simulink library "PTOSim_Lib_UpdatedV3"  (R2020b)
settings: Solver=ode45  StartTime=0.0  StopTime=10.0  RelTol=1e-3  EnableMultiTasking=on
undefined symbols (not defined in the file or in its folder): DiscIntNeverNeededParam, ptosim, PTOSimBlock, simu
libraries: $bdroot x6
(part 1 of 2)
settings Model: RequirementInfo="{}  %GIDa_42666abb_d6d9_408c_ae24_f6520282b61c"  Creator=sor  LastModifiedBy=jleonqu
settings DataIOCC: LimitDataPoints=on  SaveFormat=Array  ReturnWorkspaceOutputs=off
settings OptimizationCC: LifeSpan=inf
settings DebuggingCC: SolverPrmCheckMsg=warning  AllowSymbolicDim=off  SFUnexpectedBacktrackingDiag=warning  SFNoUnconditionalDefaultTransitionDiag=warning  SFExecutionAtInitializationDiag=none  ArithmeticOperatorsInVariantConditions=warning
settings HardwareCC: ProdBitPerPointer=32  ProdBitPerSizeT=32  ProdBitPerPtrDiffT=32  ProdLargestAtomicFloat=None  ProdIntDivRoundTo=Undefined  ProdEndianess=Unspecified  ProdWordSize=32  ProdHWDeviceType=32-bit Generic
settings ModelReferenceCC: PropagateSignalLabelsOutOfModel=off
settings SFSimCC: SimUseLocalCustomCode=off  CustomCodeUndefinedFunction=UseInterfaceOnly
settings RTWCC: RTWUseLocalCustomCode=off
settings CodeAppCC: StateflowObjectComments=on
settings GRTTargetCC: TargetLangStandard=C89/C90 (ANSI)
settings ConfigComp: CovMetricSettings=dw  CovSaveCumulativeToWorkspaceVar=on  CovSaveSingleToWorkspaceVar=on  CovExternalEMLEnable=off  CovSFcnEnable=off

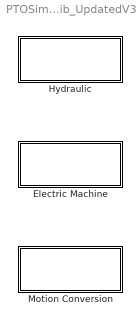
== system PTOSim_Lib_UpdatedV3 ==
  Electric Machine : Subsystem  RequirementInfo="{}  %GIDa_5439fdb4_7c29_433c_8677_23bf92e18f11"
  Hydraulic : Subsystem  RequirementInfo={} %GIDa_f12a42eb_b9cb_4818_b573_b7dee4183a3b
  Motion Conversion : Subsystem

== system PTOSim_Lib_UpdatedV3/Electric Machine ==
  Electric Machine Equivalent Circuit : Subsystem  mask{PTOSimBlock=PTOSimBlock(1), InputFiletext=Use PTO-Sim input file to define Electric Machine parameters, Ra=0, La=0, Ke=0, bShaft=0, Jem=0}
      mask prompts: PTOSimBlock "Electric Machine Name"; Ra "Armature Resistance [ohm]"; La "Armature Inductance [H]"; Ke "Back-emf or Torque constant [V/(rad/s)]"; bShaft "Rotor Damping [N s/m]"; Jem "Rotor Inertia [kg m^2]"
      mask init:
      | if exist('PTOSimBlock','var')
      |     h=[gcb '/To Workspace'];
      |     responseName=['PTOSimBlock' num2str(PTOSimBlock.PTOSimBlockNum) '_out'];
      |     set_param(h,'VariableName',responseName);
      | end
      | clear h responseName
      | %HydraulicBlock.checkLoc('W');
      settings: PortSchema="{\"entries\":[{\"content\":{\"sides\":[{\"content\":{\"connectorIds\":[\"In1\"]},\"type\":\"ConnectorPlacement.EquallySpacedRectSide\",\"uuid\":\"38b15b7d-d952-45b6-9eb0-5d473736364e\"},{\"content\":{\"connectorIds\":[\"Out1\"],\"side\":\"RIGHT\"},\"type\":\"ConnectorPlacement.EquallySpacedRectSide\",\"uuid\":\"de64adb9-f2de-4dd5-b519-c63af884483d\"},{\"content\":{\"connectorIds\":[\"In2\"],\"side\":\"TOP\"},\"type\":\"ConnectorPlacement.EquallySpacedRectSide\",\"uuid\":\"eaa9506a-5e37-41b4-975c-a8d526700d36\"},{\"content\":{\"connectorIds\":[],\"side\":\"HIDDEN\"},\"type\":\"ConnectorPlacement.EquallySpacedRectSide\",\"uuid\":\"f8da1221-e5bc-4844-b966-beaaa1d6bf60\"}]},\"type\":\"ConnectorPlacement.EquallySpacedConnector\",\"uuid\":\"4da2b473-e94d-42dc-9143-64fbcbf5d9e1\"}],\"packageUris\":[\"http://schema.mathworks.com/mf0/Connector/R2020b\"],\"version\":\"1.0\"}"
      mask DialogControl ParameterGroupVar Prompt: Custom Parameters
      mask DialogControl EMParameters Prompt: Electric Machine Parameters
      mask Display: image('ElectricMotor.png'); % Use "Edit Image" on toolstrip to change.

== system PTOSim_Lib_UpdatedV3/Hydraulic ==
  Compressible Fluid Piston Updated : Subsystem  mask{PTOSimBlock=PTOSimBlock(1), InputFileText=Use PTO-Sim input file to define PTO parameters, Ap_A=0, Ap_B=0, PistonStroke=0, BulkModulus=0, xi_piston=0, pAi=0, pBi=0}
      mask prompts: PTOSimBlock "Piston Name"; Ap_A "Piston area A [m]"; Ap_B "Piston area B [m]"; PistonStroke "Piston stroke [m]"; BulkModulus "Fluid Bulk Modulus [Pa]"; xi_piston "Piston initial displacement from A [m]"; pAi "Port A Initial pressure [Pa]"; pBi "Port B Initial pressure [Pa]"
      mask help:
      | PTO-Sim Compressible Fluid Piston
      |
      | This block simualtes a hydraulic cylinder using a compressible fluid model. The block inputs are Response and HydraulicInput. Response is the signal output of the block Rotational PTO Actuation Force. HydraulicInput is a two signal vector with the information of the flow rate for port A and port B of the cylinder. The output of the block is PistonOutput, which is a three signal vector with PressureA, PressureB, and ForcePTO.
      mask init: same as PTOSim_Lib_UpdatedV3/Electric Machine/Electric Machine Equivalent Circuit
      settings: PortSchema="{\"entries\":[{\"content\":{\"sides\":[{\"content\":{\"connectorIds\":[\"In1\"]},\"type\":\"ConnectorPlacement.EquallySpacedRectSide\",\"uuid\":\"c8df0997-125e-484b-91e1-8ba4eadd9153\"},{\"content\":{\"connectorIds\":[\"Out1\"],\"side\":\"RIGHT\"},\"type\":\"ConnectorPlacement.EquallySpacedRectSide\",\"uuid\":\"941eb644-8b58-45e1-b334-77edb1550c04\"},{\"content\":{\"connectorIds\":[\"In2\"],\"side\":\"TOP\"},\"type\":\"ConnectorPlacement.EquallySpacedRectSide\",\"uuid\":\"a73e5632-eedc-448d-9008-671742bb1d71\"},{\"content\":{\"connectorIds\":[],\"side\":\"HIDDEN\"},\"type\":\"ConnectorPlacement.EquallySpacedRectSide\",\"uuid\":\"aff918e7-82cf-4cd9-bf12-32a09e9272a3\"}]},\"type\":\"ConnectorPlacement.EquallySpacedConnector\",\"uuid\":\"3f3f511d-44ea-4688-8800-5cd126269ecd\"}],\"packageUris\":[\"http://schema.mathworks.com/mf0/Connector/R2020b\"],\"version\":\"1.0\"}"
      mask Help:
      | This block simualtes a hydraulic cylinder using a compressible fluid model. The block inputs are Response and HydraulicInput. Response is the signal output of the block Rotational PTO Actuation Force. HydraulicInput is a two signal vector with the information of the flow rate for port A and port B of the cylinder. The output of the block is PistonOutput, which is a three signal vector with PressureA, PressureB, and ForcePTO.
      | 
      | The outputs are calculated using the model presented in the following link: http://wec-sim.github.io/WEC-Sim/master/user/advanced_features.html#pto-sim
      mask DialogControl ParameterGroupVar Prompt: Custom Parameters
      mask DialogControl PistonProperties Prompt: Piston Properties
      mask DialogControl InitialConditions Prompt: Initial Conditions
      mask Display: image('DoubleActingPiston.png'); % Use "Edit Image" on toolstrip to change.
  Compressible Fluid Piston Updated Inputs : Subsystem  mask{PTOSimBlock=PTOSimBlock(1), InputFileText=Use WEC-Sim input file to define PTO parameters, Ap_A=0, Ap_B=0, PistonStroke=0, BulkModulus=0, xi_piston=0, pAi=0, pBi=0}
      mask prompts: PTOSimBlock "Piston Name"; Ap_A "Piston area A [m]"; Ap_B "Piston area B [m]"; PistonStroke "Piston stroke [m]"; BulkModulus "Fluid Bulk Modulus [Pa]"; xi_piston "Piston initial displacement from A [m]"; pAi "Port A Initial pressure [Pa]"; pBi "Port B Initial pressure [Pa]"
      mask help:
      | PTO-Sim Compressible Fluid Piston
      |
      | This block simualtes a hydraulic cylinder using a compressible fluid model. The block inputs are Response, QA and QB. Response is the signal output of the block Rotational PTO Actuation Force. QA and QB are the flow rate for port A and port B of the cylinder. The outputs of the block are ForcePTO, PA, and PB.
      mask init: same as PTOSim_Lib_UpdatedV3/Electric Machine/Electric Machine Equivalent Circuit
      settings: PortSchema="{\"entries\":[{\"content\":{\"sides\":[{\"content\":{\"connectorIds\":[\"In1\",\"In2\"]},\"type\":\"ConnectorPlacement.EquallySpacedRectSide\",\"uuid\":\"572dbc7c-8f4c-46fc-9000-663c89355fbd\"},{\"content\":{\"connectorIds\":[\"Out1\",\"Out2\",\"Out3\"],\"side\":\"RIGHT\"},\"type\":\"ConnectorPlacement.EquallySpacedRectSide\",\"uuid\":\"3b7821ce-a540-4de1-8f34-0d55375c774c\"},{\"content\":{\"connectorIds\":[\"In3\"],\"side\":\"TOP\"},\"type\":\"ConnectorPlacement.EquallySpacedRectSide\",\"uuid\":\"b6f5c275-868d-447d-b609-cdda14e9f222\"},{\"content\":{\"connectorIds\":[],\"side\":\"HIDDEN\"},\"type\":\"ConnectorPlacement.EquallySpacedRectSide\",\"uuid\":\"5b34aa5d-01fb-4d75-9f22-3e4ce64ee132\"}]},\"type\":\"ConnectorPlacement.EquallySpacedConnector\",\"uuid\":\"5b16a2f7-6624-4a26-89bf-8d87cef610e1\"}],\"packageUris\":[\"http://schema.mathworks.com/mf0/Connector/R2020b\"],\"version\":\"1.0\"}"
      mask Help:
      | This block simualtes a hydraulic cylinder using a compressible fluid model. The block inputs are Response and HydraulicInput. Response is the signal output of the block Rotational PTO Actuation Force. HydraulicInput is a two signal vector with the information of the flow rate for port A and port B of the cylinder. The output of the block is PistonOutput, which is a three signal vector with PressureA, PressureB, and ForcePTO.
      | 
      | The outputs are calculated using the model presented in the following link: http://wec-sim.github.io/WEC-Sim/master/user/advanced_features.html#pto-sim
      mask DialogControl ParameterGroupVar Prompt: Custom Parameters
      mask DialogControl PistonProperties Prompt: Piston Properties
      mask DialogControl InitialConditions Prompt: Initial Conditions
      mask Display: image('DoubleActingPiston.png'); % Use "Edit Image" on toolstrip to change.
  Fixed Displacement Hydraulic Motor : Subsystem  mask{PTOSimBlock=PTOSimBlock(1), InputFileText=Use WEC-Sim input file to define PTO parameters, Displacement=0, EffTableDeltaP=0, EffTableShaftSpeed=0, EffTableMechEff=0, EffTableVolEff=0}
      mask prompts: PTOSimBlock "Hydraulic Motor Name"; Displacement "Displacement [cc/rev]"; EffTableDeltaP "Pressure data [Pa]"; EffTableShaftSpeed "Shaft Speed Data [rpm]"; EffTableMechEff "Mechanical Efficiency"; EffTableVolEff "Volumetric Efficiency"
      mask init: same as PTOSim_Lib_UpdatedV3/Electric Machine/Electric Machine Equivalent Circuit
      mask DialogControl ParameterGroupVar Prompt: Custom Parameters
      mask DialogControl HMProperties Prompt: Hydraulic Motor Properties
      mask Display: image('FixedHydraulicMotor.png'); % Use "Edit Image" on toolstrip to change.
  Gas-Charged Hydraulic Accumulator : Subsystem  mask{PTOSimBlock=PTOSimBlock(1), InputFileText=Use PTO-Sim input file to define PTO parameters, VI0=0, VIeq=0, pIprecharge=0}
      mask prompts: PTOSimBlock "Accumulator Name"; VI0 "Total Volume [m^3]"; VIeq "Initial Volume [m^3]"; pIprecharge "Precharge [Pa]"
      mask init: same as PTOSim_Lib_UpdatedV3/Electric Machine/Electric Machine Equivalent Circuit
      mask DialogControl ParameterGroupVar Prompt: Custom Parameters
      mask DialogControl AccProperties Prompt: Accumulator Properties
      mask Display: image('GasAccumulator.png'); % Use "Edit Image" on toolstrip to change.
  Rectifying Check Valve : Subsystem  mask{PTOSimBlock=PTOSimBlock(1), InputFileText=Use PTO-Sim input file to define PTO parameters, Cd=0, Amax=0, Amin=0, pMin=0, pMax=0, rho=0, k1=0, k2=0}
      mask prompts: PTOSimBlock "Rectifying Valve Name"; Cd "Discharge coefficient"; Amax "Maximum opening area"; Amin "Minimum opening Area"; pMin "Cracking pressure"; pMax "Pressure at maximum opening"; rho "Fluid density"; k1 "Valve Coefficient k1"; k2 "Valve Coefficient k2"
      mask init: same as PTOSim_Lib_UpdatedV3/Electric Machine/Electric Machine Equivalent Circuit
      mask DialogControl ParameterGroupVar Prompt: Custom Parameters
      mask DialogControl CheckValveProperties Prompt: Check valve properties
      mask Display: image('RectifyingCheckValve.png'); % Use "Edit Image" on toolstrip to change.

== system PTOSim_Lib_UpdatedV3/Motion Conversion ==
  Rotary to Linear Adjustable Rod : Subsystem  mask{ptosim=ptosim.motionMechanism(1)}
      mask prompts: ptosim "Telescope Name:"
      mask init:
      | if exist('ptosim','var')
      |     h = [gcb '/To Workspace'];
      |     responseName = ['motionMechanism' num2str(ptosim.number) '_out'];
      |     set_param(h,'VariableName',responseName);
      |     if ischar(ptosim.crank)==1 ...
      |             || ischar(ptosim.rodInit)==1 ...
      |             || ischar(ptosim.offset)==1 ...
      |             error('One of the rotary to linear adjustable rod variables is undefined. For example, ptosim.motionMechanism.variableName')
      |     end
      | end
      | clear h responseName
  Rotary to Linear Crank : Subsystem  mask{ptosim=ptosim.motionMechanism(1)}
      mask prompts: ptosim "Crank Name:"
      mask init:
      | if exist('ptosim','var')
      |     h = [gcb '/To Workspace'];
      |     responseName = ['motionMechanism' num2str(ptosim.number) '_out'];
      |     set_param(h,'VariableName',responseName);
      |     if ischar(ptosim.crank)==1 ...
      |             || ischar(ptosim.rodLength)==1 ...
      |             || ischar(ptosim.offset)==1 ...
      |             error('One of the rotary to linear crank variables is undefined. For example, ptosim.motionMechanism.variableName')
      |     end
      | end
      | clear h responseName

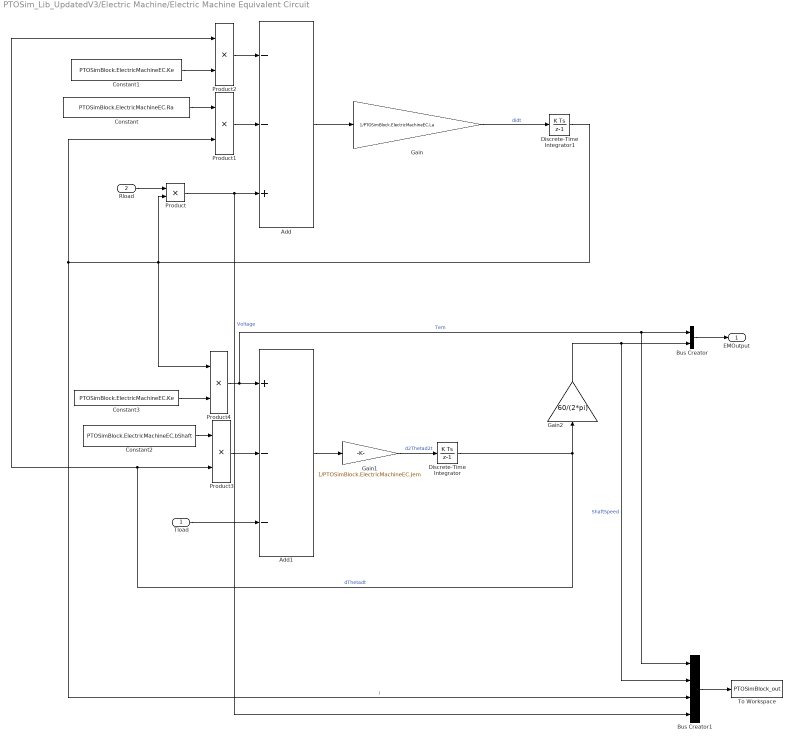
== system PTOSim_Lib_UpdatedV3/Electric Machine/Electric Machine Equivalent Circuit ==
  Tload : Inport
  Rload : Inport  Port=2
  Add : Sum  Inputs=--+
  Add1 : Sum  Inputs=+--
  Bus Creator : BusCreator  Inputs=2
  Bus Creator1 : BusCreator  Inputs=4
  Constant : Constant  Value=PTOSimBlock.ElectricMachineEC.Ra
  Constant1 : Constant  Value=PTOSimBlock.ElectricMachineEC.Ke
  Constant2 : Constant  Value=PTOSimBlock.ElectricMachineEC.bShaft
  Constant3 : Constant  Value=PTOSimBlock.ElectricMachineEC.Ke
  Discrete-Time Integrator : DiscreteIntegrator  SampleTime=-1  ICPrevOutput=DiscIntNeverNeededParam  ICPrevScaledInput=DiscIntNeverNeededParam
  Discrete-Time Integrator1 : DiscreteIntegrator  SampleTime=-1  ICPrevOutput=DiscIntNeverNeededParam  ICPrevScaledInput=DiscIntNeverNeededParam
  Gain : Gain  Gain=1/PTOSimBlock.ElectricMachineEC.La
  Gain1 : Gain  Gain=1/PTOSimBlock.ElectricMachineEC.Jem
  Gain2 : Gain  Gain=60/(2*pi)
  Product{,1..4} (5 alike) : Product
  To Workspace : ToWorkspace  VariableName=PTOSimBlock_out  SaveFormat=Timeseries  SampleTime=simu.dtOut
  EMOutput : Outport
  wires:
  Add/1 -> Gain/1
  Gain/1 -> Discrete-Time Integrator1/1  "didt"
  Rload/1 -> Product/1
  Discrete-Time Integrator1/1 -> Product4/1, Product/2, Bus Creator1/3, Product1/2  "i"
  Product/1 -> Bus Creator1/4, Add/3  "Voltage"
  Product1/1 -> Add/2
  Constant/1 -> Product1/1
  Product2/1 -> Add/1
  Constant1/1 -> Product2/2
  Tload/1 -> Add1/3
  Add1/1 -> Gain1/1
  Gain1/1 -> Discrete-Time Integrator/1  "d2Thetad2t"
  Product3/1 -> Add1/2
  Constant2/1 -> Product3/1
  Discrete-Time Integrator/1 -> Product2/1, Product3/2, Gain2/1  "dThetadt"
  Product4/1 -> Bus Creator1/1, Bus Creator/1, Add1/1  "Tem"
  Constant3/1 -> Product4/2
  Bus Creator/1 -> EMOutput/1
  Gain2/1 -> Bus Creator1/2, Bus Creator/2  "ShaftSpeed"
  Bus Creator1/1 -> To Workspace/1

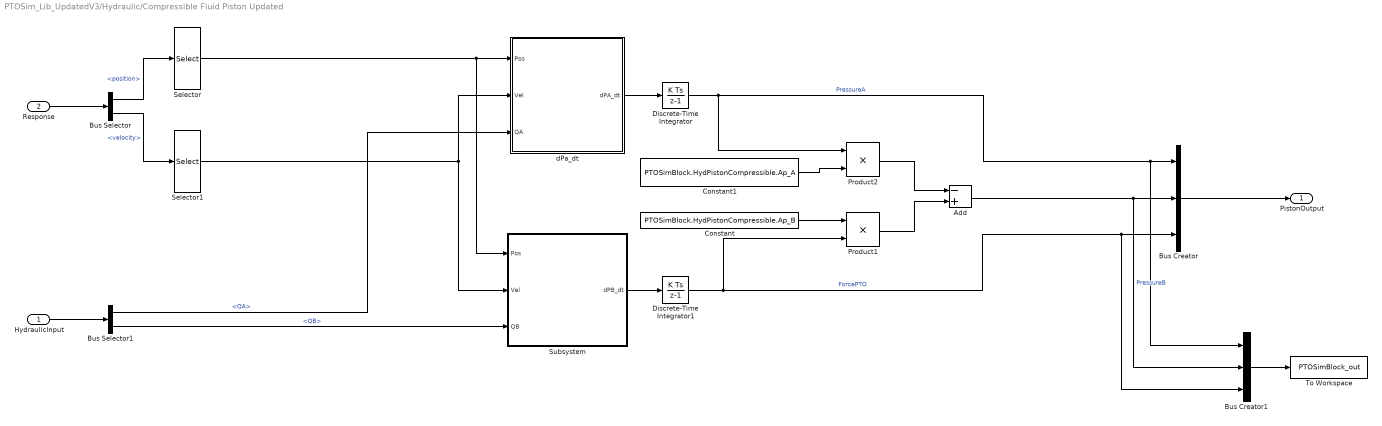
== system PTOSim_Lib_UpdatedV3/Hydraulic/Compressible Fluid Piston Updated ==
  HydraulicInput : Inport
  Response : Inport  Port=2
  Add : Sum  Inputs=-+
  Bus Creator : BusCreator  Inputs=3
  Bus Creator1 : BusCreator  Inputs=3
  Bus Selector : BusSelector  OutputSignals=position,velocity
  Bus Selector1 : BusSelector  OutputSignals=QA,QB
  Constant : Constant  Value=PTOSimBlock.HydPistonCompressible.Ap_B
  Constant1 : Constant  Value=PTOSimBlock.HydPistonCompressible.Ap_A
  Discrete-Time Integrator : DiscreteIntegrator  InitialCondition=PTOSimBlock.HydPistonCompressible.pAi  SampleTime=-1  ICPrevOutput=DiscIntNeverNeededParam  ICPrevScaledInput=DiscIntNeverNeededParam
  Discrete-Time Integrator1 : DiscreteIntegrator  InitialCondition=PTOSimBlock.HydPistonCompressible.pBi  SampleTime=-1  ICPrevOutput=DiscIntNeverNeededParam  ICPrevScaledInput=DiscIntNeverNeededParam
  Product1 : Product
  Product2 : Product
  Selector : Selector  InputPortWidth=6  IndexOptions=Index vector (dialog)  Indices=3  OutputSizes=1
  Selector1 : Selector  InputPortWidth=6  IndexOptions=Index vector (dialog)  Indices=3  OutputSizes=1
  Subsystem : Subsystem  AncestorBlock=PTOSim_Lib_Updated/Hydraulic/Compressible Fluid Piston Updated/Subsystem
  To Workspace : ToWorkspace  VariableName=PTOSimBlock_out  SaveFormat=Structure With Time  SampleTime=simu.dtOut
  dPa_dt : Subsystem  AncestorBlock=PTOSim_Lib_Updated/Hydraulic/Compressible Fluid Piston Updated/dPa_dt
  PistonOutput : Outport
  wires:
  Bus Selector/1 -> Selector/1  "<position>"
  Product1/1 -> Add/2
  HydraulicInput/1 -> Bus Selector1/1
  Subsystem/1(dPB_dt) -> Discrete-Time Integrator1/1
  dPa_dt/1(dPA_dt) -> Discrete-Time Integrator/1
  Product2/1 -> Add/1
  Selector/1 -> Subsystem/1(Pos), dPa_dt/1(Pos)
  Discrete-Time Integrator/1 -> Bus Creator1/1, Bus Creator/1, Product2/1  "PressureA"
  Response/1 -> Bus Selector/1
  Selector1/1 -> Subsystem/2(Vel), dPa_dt/2(Vel)
  Discrete-Time Integrator1/1 -> Bus Creator1/3, Bus Creator/3, Product1/2  "ForcePTO"
  Bus Selector/2 -> Selector1/1  "<velocity>"
  Constant/1 -> Product1/1
  Constant1/1 -> Product2/2
  Add/1 -> Bus Creator1/2, Bus Creator/2  "PressureB"
  Bus Creator/1 -> PistonOutput/1
  Bus Selector1/2 -> Subsystem/3(QB)  "<QB>"
  Bus Selector1/1 -> dPa_dt/3(QA)  "<QA>"
  Bus Creator1/1 -> To Workspace/1

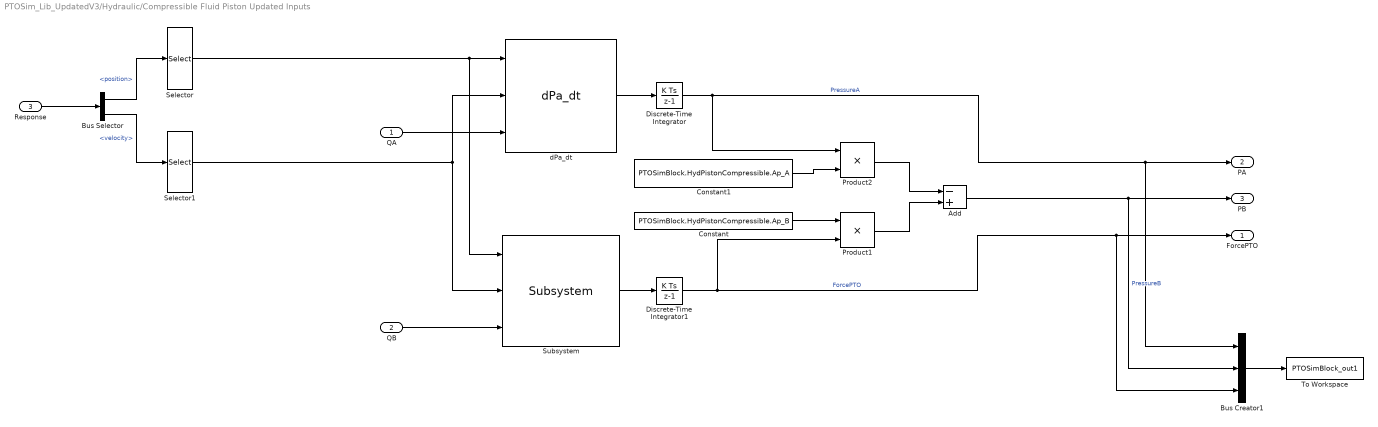
== system PTOSim_Lib_UpdatedV3/Hydraulic/Compressible Fluid Piston Updated Inputs ==
  QA : Inport
  QB : Inport  Port=2
  Response : Inport  Port=3
  Add : Sum  Inputs=-+
  Bus Creator1 : BusCreator  Inputs=3
  Bus Selector : BusSelector  OutputSignals=position,velocity
  Constant : Constant  Value=PTOSimBlock.HydPistonCompressible.Ap_B
  Constant1 : Constant  Value=PTOSimBlock.HydPistonCompressible.Ap_A
  Discrete-Time Integrator : DiscreteIntegrator  InitialCondition=PTOSimBlock.HydPistonCompressible.pAi  SampleTime=-1  ICPrevOutput=DiscIntNeverNeededParam  ICPrevScaledInput=DiscIntNeverNeededParam
  Discrete-Time Integrator1 : DiscreteIntegrator  InitialCondition=PTOSimBlock.HydPistonCompressible.pBi  SampleTime=-1  ICPrevOutput=DiscIntNeverNeededParam  ICPrevScaledInput=DiscIntNeverNeededParam
  Product1 : Product
  Product2 : Product
  Selector : Selector  InputPortWidth=6  IndexOptions=Index vector (dialog)  Indices=3  OutputSizes=1
  Selector1 : Selector  InputPortWidth=6  IndexOptions=Index vector (dialog)  Indices=3  OutputSizes=1
  Subsystem : $bdroot/Hydraulic/Compressible Fluid Piston Updated/Subsystem  SystemSampleTime=-1  VariantActivationTime=update diagram  Latency=0  AutoFrameSizeCalculation=off
  To Workspace : ToWorkspace  VariableName=PTOSimBlock_out1  SaveFormat=Structure With Time  SampleTime=simu.dtOut
  dPa_dt : $bdroot/Hydraulic/Compressible Fluid Piston Updated/dPa_dt  SystemSampleTime=-1  VariantActivationTime=update diagram  Latency=0  AutoFrameSizeCalculation=off
  ForcePTO : Outport
  PA : Outport  Port=2
  PB : Outport  Port=3
  wires:
  QA/1 -> dPa_dt/3
  Constant1/1 -> Product2/2
  Discrete-Time Integrator1/1 -> ForcePTO/1, Bus Creator1/3, Product1/2  "ForcePTO"
  Selector/1 -> Subsystem/1, dPa_dt/1
  Add/1 -> Bus Creator1/2, PB/1  "PressureB"
  Bus Creator1/1 -> To Workspace/1
  QB/1 -> Subsystem/3
  Product1/1 -> Add/2
  dPa_dt/1 -> Discrete-Time Integrator/1
  Product2/1 -> Add/1
  Constant/1 -> Product1/1
  Bus Selector/2 -> Selector1/1  "<velocity>"
  Subsystem/1 -> Discrete-Time Integrator1/1
  Selector1/1 -> Subsystem/2, dPa_dt/2
  Response/1 -> Bus Selector/1
  Discrete-Time Integrator/1 -> PA/1, Bus Creator1/1, Product2/1  "PressureA"
  Bus Selector/1 -> Selector/1  "<position>"

== system PTOSim_Lib_UpdatedV3/Hydraulic/Fixed Displacement Hydraulic Motor ==
  DeltaP : Inport
  Shaft Speed : Inport  Port=2
  Constant : Constant  Value=PTOSimBlock.HydraulicMotor.Displacement
  Constant1 : Constant  Value=PTOSimBlock.HydraulicMotor.Displacement
  Divide : Product  Inputs=/*
  Gain : Gain  Gain=1/((100^3)*2*pi)
  Gain1 : Gain  Gain=1/((100^3)*60)
  MechanicalEfficiency : Lookup_n-D  BreakpointsForDimension1=PTOSimBlock.HydraulicMotor.EffTableShaftSpeed  BreakpointsForDimension2=PTOSimBlock.HydraulicMotor.EffTableDeltaP  Table=PTOSimBlock.HydraulicMotor.EffTableMechEff  InternalRulePriority=Speed  RndMeth=Simplest  InputSameDT=on
      settings: InputPortMap=u0,u1
  Product : Product
  Product1 : Product  Inputs=3
  VolumetricEfficiency : Lookup_n-D  BreakpointsForDimension1=PTOSimBlock.HydraulicMotor.EffTableShaftSpeed  BreakpointsForDimension2=PTOSimBlock.HydraulicMotor.EffTableDeltaP  Table=PTOSimBlock.HydraulicMotor.EffTableVolEff  InternalRulePriority=Speed  RndMeth=Simplest  InputSameDT=on
      settings: InputPortMap=u0,u1
  Torque : Outport
  FlowRate : Outport  Port=2
  wires:
  DeltaP/1 -> Product1/2, VolumetricEfficiency/1, MechanicalEfficiency/1
  Shaft Speed/1 -> MechanicalEfficiency/2, Product/1, VolumetricEfficiency/2
  MechanicalEfficiency/1 -> Product1/3
  Constant/1 -> Gain/1
  Gain/1 -> Product1/1
  Product1/1 -> Torque/1
  VolumetricEfficiency/1 -> Divide/1
  Product/1 -> Divide/2
  Divide/1 -> FlowRate/1
  Constant1/1 -> Gain1/1
  Gain1/1 -> Product/2

== system PTOSim_Lib_UpdatedV3/Hydraulic/Gas-Charged Hydraulic Accumulator ==
  FlowRate : Inport
  Add1 : Sum  Inputs=-+
  Bus Creator : BusCreator  Inputs=2
  Constant4 : Constant  Value=PTOSimBlock.GasHydAccumulator.pIprecharge
  Constant5 : Constant  Value=PTOSimBlock.GasHydAccumulator.VI0
  Constant6 : Constant  Value=PTOSimBlock.GasHydAccumulator.VI0
  Constant7 : Constant  Value=1.4
  Discrete-Time Integrator1 : DiscreteIntegrator  SampleTime=-1  ICPrevOutput=DiscIntNeverNeededParam  ICPrevScaledInput=DiscIntNeverNeededParam
  Divide2 : Product  Inputs=*/
  Math Function1 : Math  Operator=pow  SaturateOnIntegerOverflow=on
  Product : Product
  To Workspace : ToWorkspace  VariableName=PTOSimBlock_out  SaveFormat=Timeseries  SampleTime=simu.dtOut
  Pressure : Outport
  wires:
  Constant4/1 -> Product/1
  Constant5/1 -> Divide2/1
  Constant6/1 -> Add1/2
  Discrete-Time Integrator1/1 -> Add1/1
  FlowRate/1 -> Bus Creator/2, Discrete-Time Integrator1/1  "FlowRate"
  Add1/1 -> Divide2/2
  Divide2/1 -> Math Function1/1
  Constant7/1 -> Math Function1/2
  Math Function1/1 -> Product/2
  Product/1 -> Bus Creator/1, Pressure/1  "Pressure"
  Bus Creator/1 -> To Workspace/1

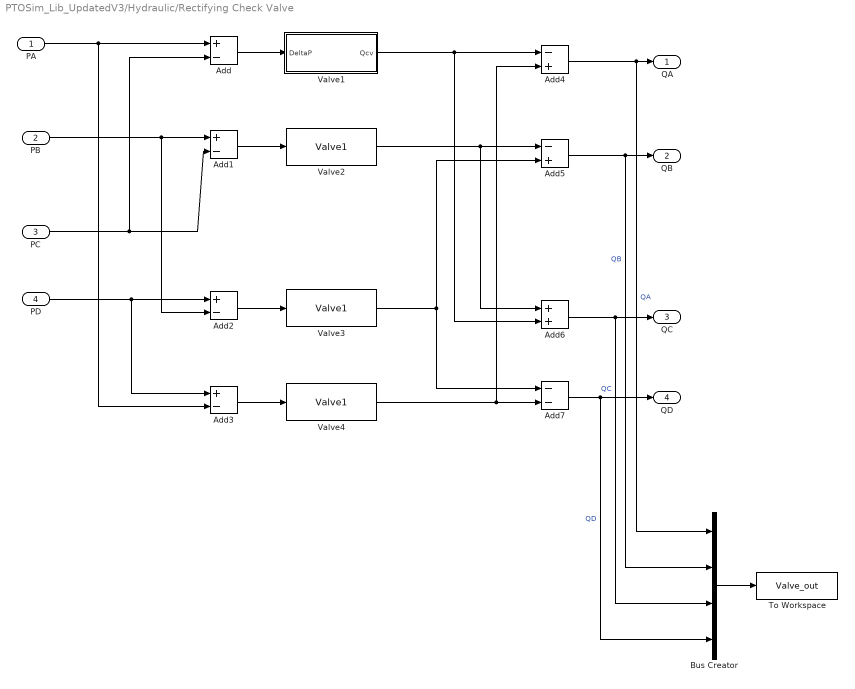
== system PTOSim_Lib_UpdatedV3/Hydraulic/Rectifying Check Valve ==
  PA : Inport
  PB : Inport  Port=2
  PC : Inport  Port=3
  PD : Inport  Port=4
  Add{,1..3} (4 alike) : Sum  Inputs=+-
  Add4 : Sum  Inputs=-+
  Add5 : Sum  Inputs=-+
  Add6 : Sum
  Add7 : Sum  Inputs=--
  Bus Creator : BusCreator  Inputs=4
  To Workspace : ToWorkspace  VariableName=Valve_out  SaveFormat=Timeseries  SampleTime=-1
  Valve1 : Subsystem
  Valve2 : $bdroot/Hydraulic/Rectifying Check Valve/Valve1  SystemSampleTime=-1  VariantActivationTime=update diagram  Latency=0  AutoFrameSizeCalculation=off
  Valve3 : $bdroot/Hydraulic/Rectifying Check Valve/Valve1  SystemSampleTime=-1  VariantActivationTime=update diagram  Latency=0  AutoFrameSizeCalculation=off
  Valve4 : $bdroot/Hydraulic/Rectifying Check Valve/Valve1  SystemSampleTime=-1  VariantActivationTime=update diagram  Latency=0  AutoFrameSizeCalculation=off
  QA : Outport
  QB : Outport  Port=2
  QC : Outport  Port=3
  QD : Outport  Port=4
  wires:
  Add/1 -> Valve1/1(DeltaP)
  PA/1 -> Add3/2, Add/1
  PC/1 -> Add/2, Add1/2
  Add1/1 -> Valve2/1
  PB/1 -> Add2/2, Add1/1
  Add2/1 -> Valve3/1
  PD/1 -> Add3/1, Add2/1
  Add3/1 -> Valve4/1
  Valve1/1(Qcv) -> Add6/2, Add4/1
  Valve4/1 -> Add7/2, Add4/2
  Valve2/1 -> Add6/1, Add5/1
  Valve3/1 -> Add7/1, Add5/2
  Add7/1 -> Bus Creator/4, QD/1  "QD"
  Add6/1 -> Bus Creator/3, QC/1  "QC"
  Add5/1 -> Bus Creator/2, QB/1  "QB"
  Bus Creator/1 -> To Workspace/1
  Add4/1 -> Bus Creator/1, QA/1  "QA"

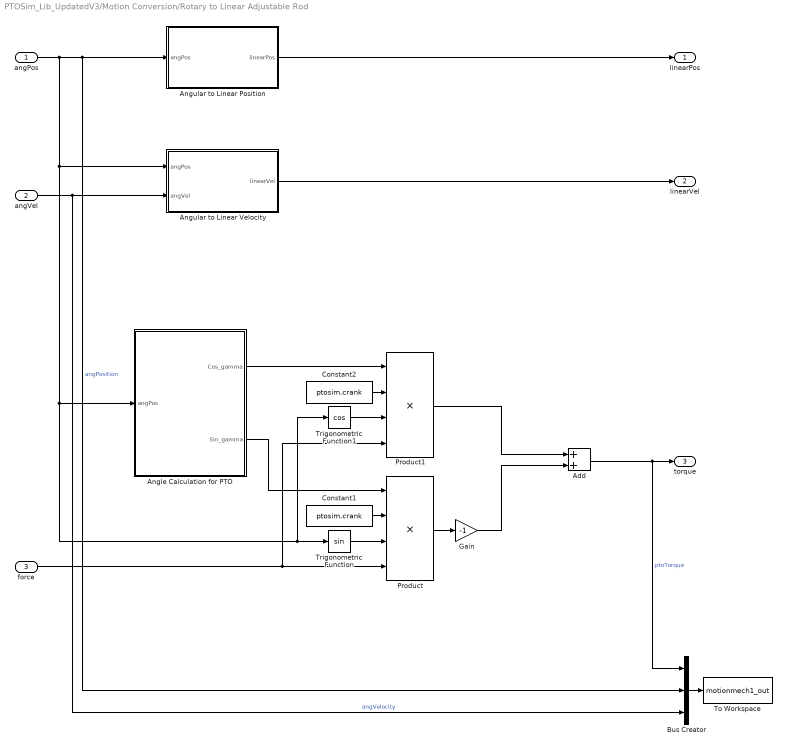
== system PTOSim_Lib_UpdatedV3/Motion Conversion/Rotary to Linear Adjustable Rod ==
  angPos : Inport
  angVel : Inport  Port=2
  force : Inport  Port=3
  Add : Sum
  Angle Calculation for PTO : Subsystem
  Angular to Linear Position : Subsystem
  Angular to Linear Velocity : Subsystem
  Bus Creator : BusCreator  Inputs=3
  Constant1 : Constant  Value=ptosim.crank
  Constant2 : Constant  Value=ptosim.crank
  Gain : Gain  Gain=-1
  Product : Product  Inputs=4
  Product1 : Product  Inputs=4
  To Workspace : ToWorkspace  VariableName=motionmech1_out  SaveFormat=Structure With Time  SampleTime=-1
      settings: Decimation=round(simu.dtOut/simu.dt,0)
  Trigonometric Function : Trigonometry
  Trigonometric Function1 : Trigonometry  Operator=cos
  linearPos : Outport
  linearVel : Outport  Port=2
  torque : Outport  Port=3
  wires:
  Angular to Linear Position/1(linearPos) -> linearPos/1
  angVel/1 -> Bus Creator/3, Angular to Linear Velocity/2(angVel)  "angVelocity"
  Angular to Linear Velocity/1(linearVel) -> linearVel/1
  Add/1 -> Bus Creator/1, torque/1  "ptoTorque"
  Bus Creator/1 -> To Workspace/1
  angPos/1 -> Angular to Linear Velocity/1(angPos), Trigonometric Function1/1, Trigonometric Function/1, Angle Calculation for PTO/1(angPos), Bus Creator/2, Angular to Linear Position/1(angPos)  "angPosition"
  Product1/1 -> Add/1
  Gain/1 -> Add/2
  Angle Calculation for PTO/2(Sin_gamma) -> Product/1
  Trigonometric Function1/1 -> Product1/3
  Angle Calculation for PTO/1(Cos_gamma) -> Product1/1
  force/1 -> Product1/4, Product/4
  Constant2/1 -> Product1/2
  Trigonometric Function/1 -> Product/3
  Constant1/1 -> Product/2
  Product/1 -> Gain/1

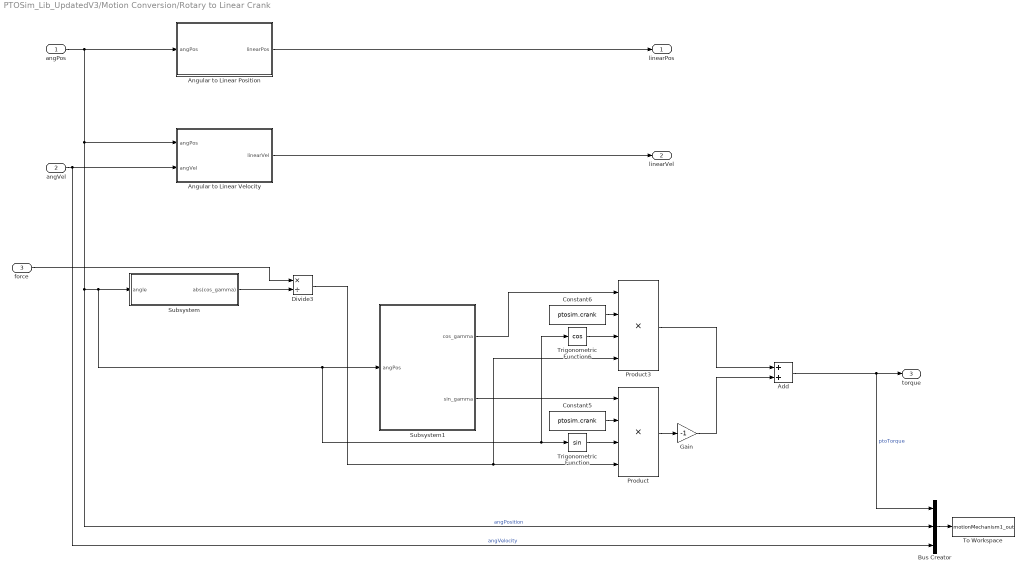
== system PTOSim_Lib_UpdatedV3/Motion Conversion/Rotary to Linear Crank ==
  angPos : Inport
  angVel : Inport  Port=2
  force : Inport  Port=3
  Add : Sum
  Angular to Linear Position : Subsystem
  Angular to Linear Velocity : Subsystem
  Bus Creator : BusCreator  Inputs=3
  Constant5 : Constant  Value=ptosim.crank
  Constant6 : Constant  Value=ptosim.crank
  Divide3 : Product  Inputs=*/
  Gain : Gain  Gain=-1
  Product : Product  Inputs=4
  Product3 : Product  Inputs=4
  Subsystem : Subsystem
  Subsystem1 : Subsystem  AncestorBlock=PTOSim_Lib/Motion Conversion/Rotary to Linear Adjustable Rod/Subsystem
  To Workspace : ToWorkspace  VariableName=motionMechanism1_out  SaveFormat=Structure With Time  SampleTime=-1
      settings: Decimation=round(simu.dtOut/simu.dt,0)
  Trigonometric Function : Trigonometry
  Trigonometric Function6 : Trigonometry  Operator=cos
  linearPos : Outport
  linearVel : Outport  Port=2
  torque : Outport  Port=3
  wires:
  Angular to Linear Position/1(linearPos) -> linearPos/1
  angVel/1 -> Bus Creator/3, Angular to Linear Velocity/2(angVel)  "angVelocity"
  Angular to Linear Velocity/1(linearVel) -> linearVel/1
  Add/1 -> Bus Creator/1, torque/1  "ptoTorque"
  Bus Creator/1 -> To Workspace/1
  Subsystem/1(abs(cos_gamma)) -> Divide3/2
  force/1 -> Divide3/1
  Trigonometric Function6/1 -> Product3/3
  Subsystem1/1(cos_gamma) -> Product3/1
  Constant6/1 -> Product3/2
  Divide3/1 -> Product/4, Product3/4
  Gain/1 -> Add/2
  Product3/1 -> Add/1
  Subsystem1/2(sin_gamma) -> Product/1
  angPos/1 -> Angular to Linear Velocity/1(angPos), Subsystem1/1(angPos), Trigonometric Function/1, Trigonometric Function6/1, Subsystem/1(angle), Bus Creator/2, Angular to Linear Position/1(angPos)  "angPosition"
  Trigonometric Function/1 -> Product/3
  Constant5/1 -> Product/2
  Product/1 -> Gain/1

== system PTOSim_Lib_UpdatedV3/Hydraulic/Compressible Fluid Piston Updated/Subsystem ==
  Pos : Inport
  Vel : Inport  Port=2
  QB : Inport  Port=3
  Add : Sum
  Add1 : Sum  Inputs=--+
  Constant : Constant  Value=PTOSimBlock.HydPistonCompressible.Ap_B
  Constant1 : Constant  Value=PTOSimBlock.HydPistonCompressible.PistonStroke
  Constant2 : Constant  Value=PTOSimBlock.HydPistonCompressible.Ap_B
  Constant3 : Constant  Value=PTOSimBlock.HydPistonCompressible.BulkModulus
  Constant4 : Constant  Value=PTOSimBlock.HydPistonCompressible.xi_piston
  Divide : Product  Inputs=/*
  Product : Product
  Product1 : Product
  Product2 : Product
  Saturation : Saturate  UpperLimit=inf  LowerLimit=1e-12
  dPB_dt : Outport
  wires:
  Constant4/1 -> Add1/2
  Constant1/1 -> Add1/3
  Product1/1 -> dPB_dt/1
  Divide/1 -> Product1/1
  Constant3/1 -> Divide/2
  Product2/1 -> Saturation/1
  Constant2/1 -> Product2/2
  Add1/1 -> Product2/1
  Pos/1 -> Add1/1
  Add/1 -> Product1/2
  QB/1 -> Add/2
  Product/1 -> Add/1
  Constant/1 -> Product/2
  Vel/1 -> Product/1
  Saturation/1 -> Divide/1

== system PTOSim_Lib_UpdatedV3/Hydraulic/Compressible Fluid Piston Updated/dPa_dt ==
  Pos : Inport
  Vel : Inport  Port=2
  QA : Inport  Port=3
  Add : Sum  Inputs=-+
  Add1 : Sum
  Constant : Constant  Value=PTOSimBlock.HydPistonCompressible.Ap_A
  Constant1 : Constant  Value=PTOSimBlock.HydPistonCompressible.BulkModulus
  Constant2 : Constant  Value=PTOSimBlock.HydPistonCompressible.xi_piston
  Constant3 : Constant  Value=PTOSimBlock.HydPistonCompressible.Ap_A
  Divide : Product  Inputs=/*
  Divide1 : Product  Inputs=*/
  Product : Product
  Product1 : Product
  Saturation : Saturate  UpperLimit=inf  LowerLimit=1e-12
  dPA_dt : Outport
  wires:
  Constant2/1 -> Add1/1
  Add1/1 -> Saturation/1
  Pos/1 -> Add1/2
  Product/1 -> Add/1
  QA/1 -> Add/2
  Constant/1 -> Product/2
  Add/1 -> Product1/2
  Divide/1 -> dPA_dt/1
  Product1/1 -> Divide/2
  Vel/1 -> Product/1
  Saturation/1 -> Divide/1
  Constant1/1 -> Divide1/1
  Constant3/1 -> Divide1/2
  Divide1/1 -> Product1/1

== system PTOSim_Lib_UpdatedV3/Hydraulic/Rectifying Check Valve/Valve1 ==
  DeltaP : Inport
  Av : Subsystem
  Constant : Constant  Value=PTOSimBlock.RectifyingCheckValve.rho
  Divide : Product  Inputs=/*
  Gain : Gain  Gain=PTOSimBlock.RectifyingCheckValve.k1
  Gain1 : Gain  Gain=2
  Gain2 : Gain  Gain=PTOSimBlock.RectifyingCheckValve.Cd
  Product : Product
  Product1 : Product
  Sqrt : Sqrt  SaturateOnIntegerOverflow=on
  Trigonometric Function : Trigonometry  Operator=tanh
  Qcv : Outport
  wires:
  DeltaP/1 -> Gain/1, Gain1/1, Av/1(DeltaP)
  Gain/1 -> Trigonometric Function/1
  Trigonometric Function/1 -> Product/1
  Gain1/1 -> Product/2
  Product/1 -> Divide/2
  Constant/1 -> Divide/1
  Divide/1 -> Sqrt/1
  Sqrt/1 -> Gain2/1
  Gain2/1 -> Product1/1
  Av/1(Av) -> Product1/2
  Product1/1 -> Qcv/1

== system PTOSim_Lib_UpdatedV3/Motion Conversion/Rotary to Linear Adjustable Rod/Angle Calculation for PTO ==
  angPos : Inport
  Add : Sum  Inputs=+-
  Add1 : Sum  Inputs=+-
  Constant1 : Constant  Value=ptosim.crank
  Constant2 : Constant  Value=ptosim.crank
  Constant3 : Constant  Value=ptosim.offset
  Distance btw flap joint & rod joint along x-axis : $bdroot/Motion Conversion/Rotary to Linear Adjustable Rod/Angular to Linear Velocity/Subsystem/Distance btw flap joint & rod joint along x-axis  SystemSampleTime=-1  VariantActivationTime=update diagram  Latency=0  AutoFrameSizeCalculation=off
  Divide : Product  Inputs=*/
  Divide1 : Product  Inputs=*/
  Product : Product
  Product1 : Product
  Subsystem1 : Subsystem  AncestorBlock=|
      | PTOSim_Lib/Motion Conversion/Rotary to Linear
      | Adjustable Rod/Angular to Linear
      | Velocity/Subsystem
  Subsystem2 : Subsystem  AncestorBlock=|
      | PTOSim_Lib/Motion Conversion/Rotary to Linear
      | Adjustable Rod/Angular to Linear
      | Velocity/Subsystem
  Trigonometric Function : Trigonometry
  Trigonometric Function1 : Trigonometry  Operator=cos
  Cos_gamma : Outport
  Sin_gamma : Outport  Port=2
  wires:
  Trigonometric Function/1 -> Product/1
  Product/1 -> Add/1
  Distance btw flap joint & rod joint along x-axis/1 -> Add/2
  Constant2/1 -> Product/2
  Add/1 -> Divide/1
  Subsystem1/1(rodLength) -> Divide/2
  Divide/1 -> Cos_gamma/1
  Subsystem2/1(rodLength) -> Divide1/2
  Trigonometric Function1/1 -> Product1/1
  Constant1/1 -> Product1/2
  Product1/1 -> Add1/1
  Constant3/1 -> Add1/2
  Add1/1 -> Divide1/1
  angPos/1 -> Subsystem1/1(angPos), Subsystem2/1(angPos), Trigonometric Function1/1, Trigonometric Function/1
  Divide1/1 -> Sin_gamma/1

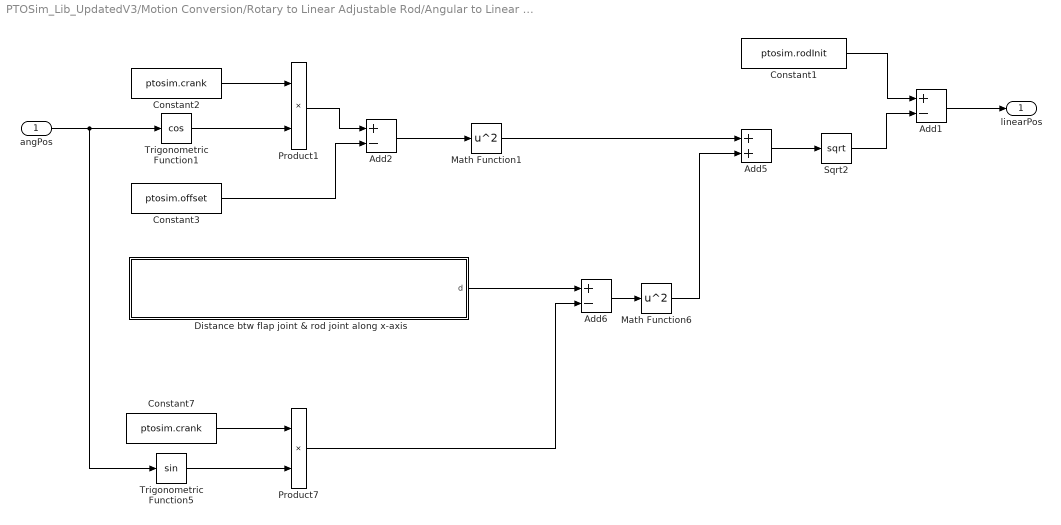
== system PTOSim_Lib_UpdatedV3/Motion Conversion/Rotary to Linear Adjustable Rod/Angular to Linear Position ==
  angPos : Inport
  Add1 : Sum  Inputs=+-
  Add2 : Sum  Inputs=+-
  Add5 : Sum
  Add6 : Sum  Inputs=+-
  Constant1 : Constant  Value=ptosim.rodInit
  Constant2 : Constant  Value=ptosim.crank
  Constant3 : Constant  Value=ptosim.offset
  Constant7 : Constant  Value=ptosim.crank
  Distance btw flap joint & rod joint along x-axis : Subsystem
  Math Function1 : Math  Operator=square  SignedPower=on  SaturateOnIntegerOverflow=on
  Math Function6 : Math  Operator=square  SignedPower=on  SaturateOnIntegerOverflow=on
  Product1 : Product  Inputs=**
  Product7 : Product  Inputs=**
  Sqrt2 : Sqrt  SaturateOnIntegerOverflow=on
  Trigonometric Function1 : Trigonometry  Operator=cos
  Trigonometric Function5 : Trigonometry
  linearPos : Outport
  wires:
  angPos/1 -> Trigonometric Function5/1, Trigonometric Function1/1
  Add1/1 -> linearPos/1
  Add2/1 -> Math Function1/1
  Trigonometric Function5/1 -> Product7/2
  Product7/1 -> Add6/2
  Add6/1 -> Math Function6/1
  Math Function6/1 -> Add5/2
  Add5/1 -> Sqrt2/1
  Sqrt2/1 -> Add1/2
  Constant1/1 -> Add1/1
  Constant2/1 -> Product1/1
  Trigonometric Function1/1 -> Product1/2
  Product1/1 -> Add2/1
  Constant3/1 -> Add2/2
  Math Function1/1 -> Add5/1
  Constant7/1 -> Product7/1
  Distance btw flap joint & rod joint along x-axis/1(d) -> Add6/1

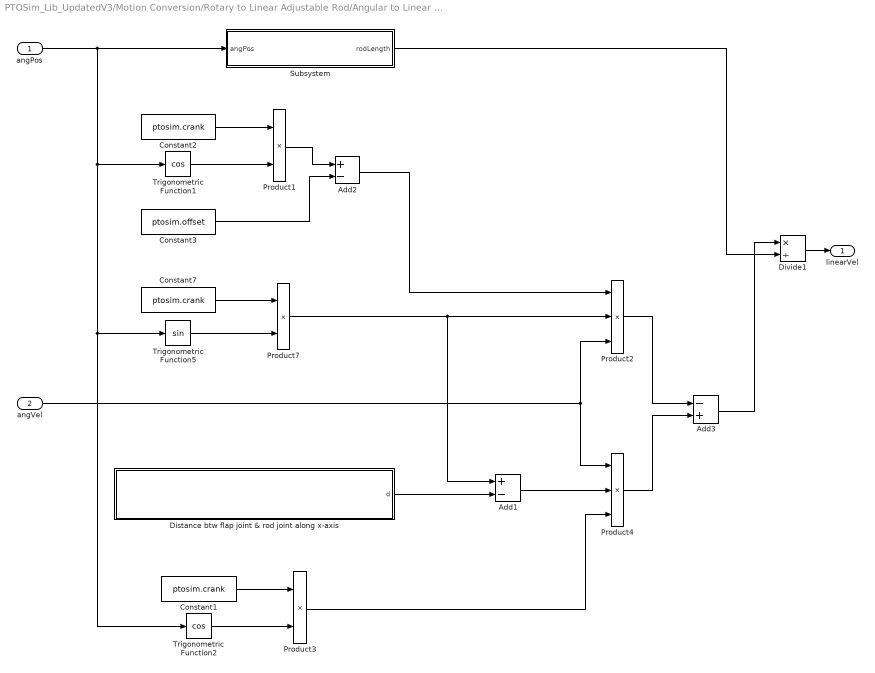
== system PTOSim_Lib_UpdatedV3/Motion Conversion/Rotary to Linear Adjustable Rod/Angular to Linear Velocity ==
  angPos : Inport
  angVel : Inport  Port=2
  Add1 : Sum  Inputs=+-
  Add2 : Sum  Inputs=+-
  Add3 : Sum  Inputs=-+
  Constant1 : Constant  Value=ptosim.crank
  Constant2 : Constant  Value=ptosim.crank
  Constant3 : Constant  Value=ptosim.offset
  Constant7 : Constant  Value=ptosim.crank
  Distance btw flap joint & rod joint along x-axis : Subsystem
  Divide1 : Product  Inputs=*/
  Product1 : Product  Inputs=**
  Product2 : Product  Inputs=***
  Product3 : Product  Inputs=**
  Product4 : Product  Inputs=***
  Product7 : Product  Inputs=**
  Subsystem : Subsystem
  Trigonometric Function1 : Trigonometry  Operator=cos
  Trigonometric Function2 : Trigonometry  Operator=cos
  Trigonometric Function5 : Trigonometry
  linearVel : Outport
  wires:
  Add2/1 -> Product2/1
  Constant2/1 -> Product1/1
  Trigonometric Function1/1 -> Product1/2
  Product1/1 -> Add2/1
  Constant3/1 -> Add2/2
  Trigonometric Function5/1 -> Product7/2
  Product7/1 -> Add1/1, Product2/2
  Constant7/1 -> Product7/1
  angVel/1 -> Product2/3, Product4/1
  Distance btw flap joint & rod joint along x-axis/1(d) -> Add1/2
  Constant1/1 -> Product3/1
  Trigonometric Function2/1 -> Product3/2
  Product3/1 -> Product4/3
  angPos/1 -> Trigonometric Function5/1, Trigonometric Function2/1, Trigonometric Function1/1, Subsystem/1(angPos)
  Add1/1 -> Product4/2
  Subsystem/1(rodLength) -> Divide1/2
  Product2/1 -> Add3/1
  Product4/1 -> Add3/2
  Add3/1 -> Divide1/1
  Divide1/1 -> linearVel/1

== system PTOSim_Lib_UpdatedV3/Motion Conversion/Rotary to Linear Crank/Angular to Linear Position ==
  angPos : Inport
  Add1 : Sum  Inputs=++-
  Add2 : Sum  Inputs=+-
  Add5 : Sum  Inputs=+-
  Constant1 : Constant  Value=ptosim.rodLength
  Constant2 : Constant  Value=ptosim.crank
  Constant3 : Constant  Value=ptosim.offset
  Constant7 : Constant  Value=ptosim.crank
  Initial Distance btw flap joint & crank joint along x-axis : Subsystem
  Math Function1 : Math  Operator=square  SignedPower=on  SaturateOnIntegerOverflow=on
  Math Function2 : Math  Operator=square  SignedPower=on  SaturateOnIntegerOverflow=on
  Product1 : Product  Inputs=**
  Product7 : Product  Inputs=**
  Sqrt2 : Sqrt  SaturateOnIntegerOverflow=on
  Trigonometric Function1 : Trigonometry  Operator=cos
  Trigonometric Function5 : Trigonometry
  linearPos : Outport
  wires:
  angPos/1 -> Trigonometric Function1/1, Trigonometric Function5/1
  Add2/1 -> Math Function1/1
  Trigonometric Function5/1 -> Product7/2
  Add5/1 -> Sqrt2/1
  Constant2/1 -> Product1/1
  Trigonometric Function1/1 -> Product1/2
  Product1/1 -> Add2/1
  Constant3/1 -> Add2/2
  Constant7/1 -> Product7/1
  Initial Distance btw flap joint & crank joint along x-axis/1(d) -> Add1/3
  Constant1/1 -> Math Function2/1
  Math Function1/1 -> Add5/2
  Sqrt2/1 -> Add1/2
  Product7/1 -> Add1/1
  Add1/1 -> linearPos/1
  Math Function2/1 -> Add5/1

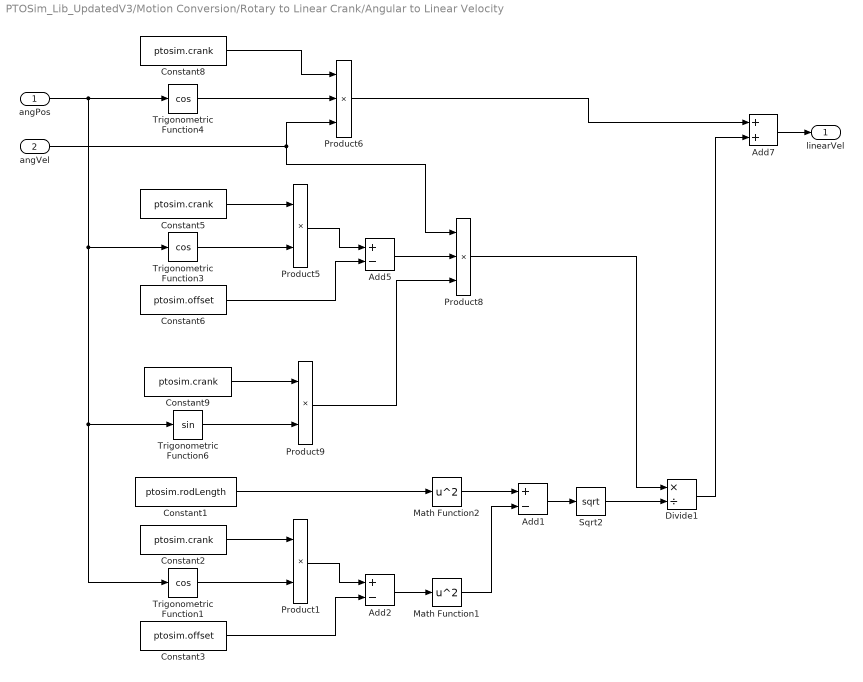
== system PTOSim_Lib_UpdatedV3/Motion Conversion/Rotary to Linear Crank/Angular to Linear Velocity ==
  angPos : Inport
  angVel : Inport  Port=2
  Add1 : Sum  Inputs=+-
  Add2 : Sum  Inputs=+-
  Add5 : Sum  Inputs=+-
  Add7 : Sum
  Constant1 : Constant  Value=ptosim.rodLength
  Constant{2,5,8..9} (4 alike) : Constant  Value=ptosim.crank
  Constant3 : Constant  Value=ptosim.offset
  Constant6 : Constant  Value=ptosim.offset
  Divide1 : Product  Inputs=*/
  Math Function1 : Math  Operator=square  SignedPower=on  SaturateOnIntegerOverflow=on
  Math Function2 : Math  Operator=square  SignedPower=on  SaturateOnIntegerOverflow=on
  Product1 : Product  Inputs=**
  Product5 : Product  Inputs=**
  Product6 : Product  Inputs=***
  Product8 : Product  Inputs=***
  Product9 : Product  Inputs=**
  Sqrt2 : Sqrt  SaturateOnIntegerOverflow=on
  Trigonometric Function1 : Trigonometry  Operator=cos
  Trigonometric Function3 : Trigonometry  Operator=cos
  Trigonometric Function4 : Trigonometry  Operator=cos
  Trigonometric Function6 : Trigonometry
  linearVel : Outport
  wires:
  Add7/1 -> linearVel/1
  Trigonometric Function4/1 -> Product6/2
  Constant8/1 -> Product6/1
  Product6/1 -> Add7/1
  Constant5/1 -> Product5/1
  Trigonometric Function3/1 -> Product5/2
  Product5/1 -> Add5/1
  Constant6/1 -> Add5/2
  Constant9/1 -> Product9/1
  Trigonometric Function6/1 -> Product9/2
  angVel/1 -> Product8/1, Product6/3
  Add5/1 -> Product8/2
  Product9/1 -> Product8/3
  angPos/1 -> Trigonometric Function1/1, Trigonometric Function6/1, Trigonometric Function3/1, Trigonometric Function4/1
  Add2/1 -> Math Function1/1
  Add1/1 -> Sqrt2/1
  Constant2/1 -> Product1/1
  Trigonometric Function1/1 -> Product1/2
  Product1/1 -> Add2/1
  Constant3/1 -> Add2/2
  Constant1/1 -> Math Function2/1
  Math Function1/1 -> Add1/2
  Sqrt2/1 -> Divide1/2
  Product8/1 -> Divide1/1
  Divide1/1 -> Add7/2
  Math Function2/1 -> Add1/1

== system PTOSim_Lib_UpdatedV3/Motion Conversion/Rotary to Linear Crank/Subsystem ==
  angle : Inport
  Add : Sum  Inputs=+-
  Add1 : Sum  Inputs=+-
  Constant : Constant
  Constant2 : Constant  Value=ptosim.crank
  Constant3 : Constant  Value=ptosim.offset
  Constant4 : Constant  Value=ptosim.rodLength
  Divide : Product  Inputs=*/
  Product : Product
  Sqrt : Sqrt  SaturateOnIntegerOverflow=on
  Square : Math  Operator=square  SignedPower=on  SaturateOnIntegerOverflow=on
  Trigonometric Function : Trigonometry  Operator=cos
  abs(cos_gamma) : Outport
  wires:
  angle/1 -> Trigonometric Function/1
  Trigonometric Function/1 -> Product/1
  Constant2/1 -> Product/2
  Product/1 -> Add/1
  Constant3/1 -> Add/2
  Add/1 -> Divide/1
  Constant4/1 -> Divide/2
  Divide/1 -> Square/1
  Square/1 -> Add1/2
  Add1/1 -> Sqrt/1
  Constant/1 -> Add1/1
  Sqrt/1 -> abs(cos_gamma)/1

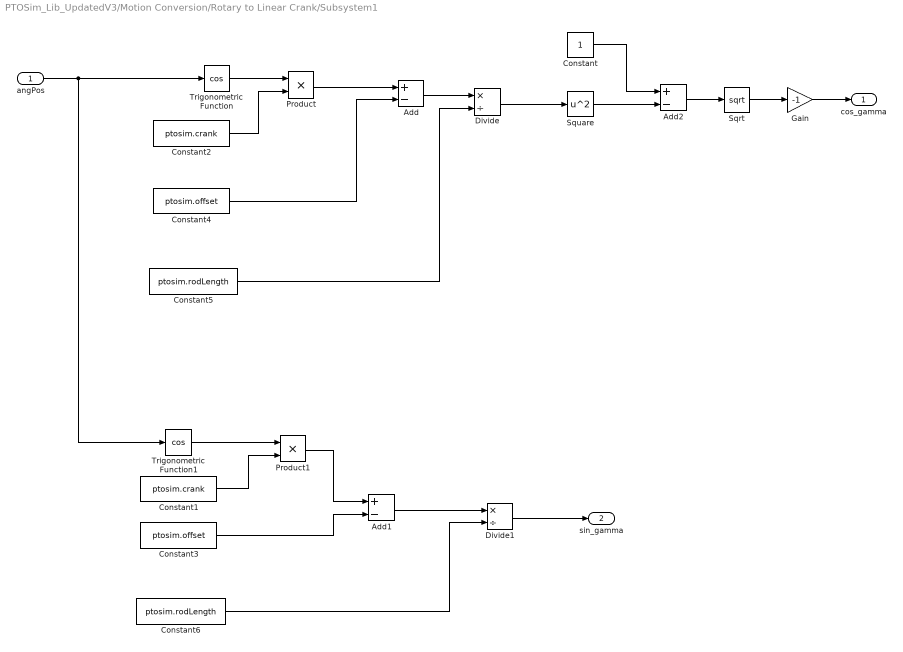
== system PTOSim_Lib_UpdatedV3/Motion Conversion/Rotary to Linear Crank/Subsystem1 ==
  angPos : Inport
  Add : Sum  Inputs=+-
  Add1 : Sum  Inputs=+-
  Add2 : Sum  Inputs=+-
  Constant : Constant
  Constant1 : Constant  Value=ptosim.crank
  Constant2 : Constant  Value=ptosim.crank
  Constant3 : Constant  Value=ptosim.offset
  Constant4 : Constant  Value=ptosim.offset
  Constant5 : Constant  Value=ptosim.rodLength
  Constant6 : Constant  Value=ptosim.rodLength
  Divide : Product  Inputs=*/
  Divide1 : Product  Inputs=*/
  Gain : Gain  Gain=-1
  Product : Product
  Product1 : Product
  Sqrt : Sqrt  SaturateOnIntegerOverflow=on
  Square : Math  Operator=square  SignedPower=on  SaturateOnIntegerOverflow=on
  Trigonometric Function : Trigonometry  Operator=cos
  Trigonometric Function1 : Trigonometry  Operator=cos
  cos_gamma : Outport
  sin_gamma : Outport  Port=2
  wires:
  Divide1/1 -> sin_gamma/1
  Add1/1 -> Divide1/1
  Constant3/1 -> Add1/2
  Product1/1 -> Add1/1
  Constant1/1 -> Product1/2
  Trigonometric Function1/1 -> Product1/1
  Constant6/1 -> Divide1/2
  Add/1 -> Divide/1
  Add2/1 -> Sqrt/1
  angPos/1 -> Trigonometric Function1/1, Trigonometric Function/1
  Square/1 -> Add2/2
  Product/1 -> Add/1
  Constant2/1 -> Product/2
  Trigonometric Function/1 -> Product/1
  Divide/1 -> Square/1
  Constant5/1 -> Divide/2
  Constant/1 -> Add2/1
  Constant4/1 -> Add/2
  Sqrt/1 -> Gain/1
  Gain/1 -> cos_gamma/1

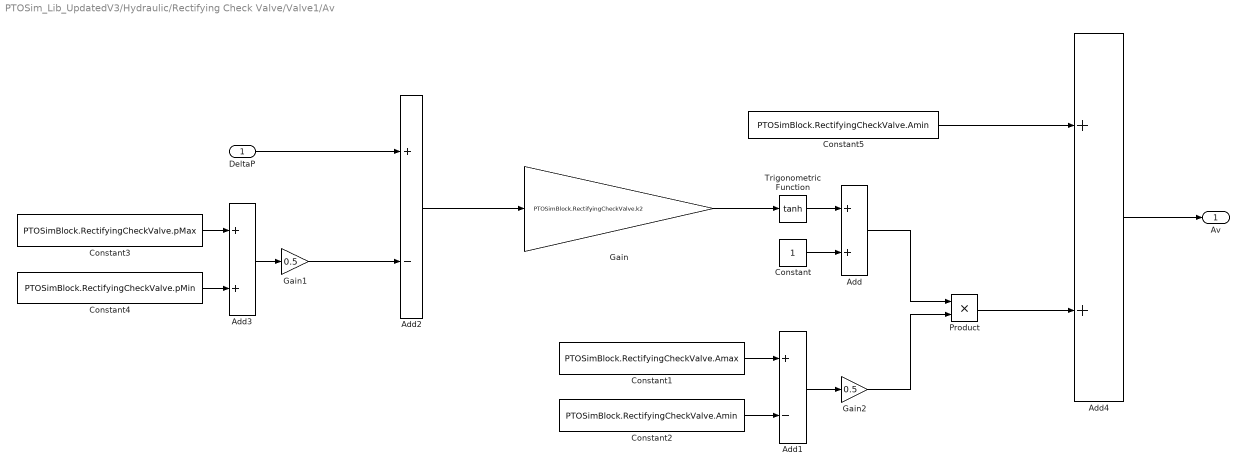
== system PTOSim_Lib_UpdatedV3/Hydraulic/Rectifying Check Valve/Valve1/Av ==
  DeltaP : Inport
  Add : Sum
  Add1 : Sum  Inputs=+-
  Add2 : Sum  Inputs=+-
  Add3 : Sum
  Add4 : Sum
  Constant : Constant
  Constant1 : Constant  Value=PTOSimBlock.RectifyingCheckValve.Amax
  Constant2 : Constant  Value=PTOSimBlock.RectifyingCheckValve.Amin
  Constant3 : Constant  Value=PTOSimBlock.RectifyingCheckValve.pMax
  Constant4 : Constant  Value=PTOSimBlock.RectifyingCheckValve.pMin
  Constant5 : Constant  Value=PTOSimBlock.RectifyingCheckValve.Amin
  Gain : Gain  Gain=PTOSimBlock.RectifyingCheckValve.k2
  Gain1 : Gain  Gain=0.5
  Gain2 : Gain  Gain=0.5
  Product : Product
  Trigonometric Function : Trigonometry  Operator=tanh
  Av : Outport
  wires:
  Constant5/1 -> Add4/1
  Product/1 -> Add4/2
  Constant3/1 -> Add3/1
  Gain/1 -> Trigonometric Function/1
  Add2/1 -> Gain/1
  Constant/1 -> Add/2
  Add1/1 -> Gain2/1
  Constant1/1 -> Add1/1
  Trigonometric Function/1 -> Add/1
  Add3/1 -> Gain1/1
  Constant2/1 -> Add1/2
  Gain1/1 -> Add2/2
  Constant4/1 -> Add3/2
  Add/1 -> Product/1
  Gain2/1 -> Product/2
  Add4/1 -> Av/1
  DeltaP/1 -> Add2/1

== system PTOSim_Lib_UpdatedV3/Motion Conversion/Rotary to Linear Adjustable Rod/Angle Calculation for PTO/Subsystem1 ==
  angPos : Inport
  Add2 : Sum  Inputs=+-
  Add5 : Sum
  Add6 : Sum  Inputs=+-
  Constant1 : Constant  Value=ptosim.crank
  Constant2 : Constant  Value=ptosim.crank
  Constant3 : Constant  Value=ptosim.offset
  Distance btw flap joint & rod joint along x-axis : Subsystem
  Math Function1 : Math  Operator=square  SignedPower=on  SaturateOnIntegerOverflow=on
  Math Function6 : Math  Operator=square  SignedPower=on  SaturateOnIntegerOverflow=on
  Product1 : Product  Inputs=**
  Product7 : Product  Inputs=**
  Sqrt2 : Sqrt  SaturateOnIntegerOverflow=on
  Trigonometric Function1 : Trigonometry  Operator=cos
  Trigonometric Function5 : Trigonometry
  rodLength : Outport
  wires:
  Distance btw flap joint & rod joint along x-axis/1(d) -> Add6/1
  Constant2/1 -> Product7/1
  Math Function1/1 -> Add5/1
  Constant3/1 -> Add2/2
  Product1/1 -> Add2/1
  Trigonometric Function1/1 -> Product1/2
  Constant1/1 -> Product1/1
  Sqrt2/1 -> rodLength/1
  Add5/1 -> Sqrt2/1
  Math Function6/1 -> Add5/2
  Add6/1 -> Math Function6/1
  Product7/1 -> Add6/2
  Trigonometric Function5/1 -> Product7/2
  Add2/1 -> Math Function1/1
  angPos/1 -> Trigonometric Function1/1, Trigonometric Function5/1

== system PTOSim_Lib_UpdatedV3/Motion Conversion/Rotary to Linear Adjustable Rod/Angle Calculation for PTO/Subsystem2 ==
  angPos : Inport
  Add2 : Sum  Inputs=+-
  Add5 : Sum
  Add6 : Sum  Inputs=+-
  Constant1 : Constant  Value=ptosim.crank
  Constant2 : Constant  Value=ptosim.crank
  Constant3 : Constant  Value=ptosim.offset
  Distance btw flap joint & rod joint along x-axis : Subsystem
  Math Function1 : Math  Operator=square  SignedPower=on  SaturateOnIntegerOverflow=on
  Math Function6 : Math  Operator=square  SignedPower=on  SaturateOnIntegerOverflow=on
  Product1 : Product  Inputs=**
  Product7 : Product  Inputs=**
  Sqrt2 : Sqrt  SaturateOnIntegerOverflow=on
  Trigonometric Function1 : Trigonometry  Operator=cos
  Trigonometric Function5 : Trigonometry
  rodLength : Outport
  wires:
  Distance btw flap joint & rod joint along x-axis/1(d) -> Add6/1
  Constant2/1 -> Product7/1
  Math Function1/1 -> Add5/1
  Constant3/1 -> Add2/2
  Product1/1 -> Add2/1
  Trigonometric Function1/1 -> Product1/2
  Constant1/1 -> Product1/1
  Sqrt2/1 -> rodLength/1
  Add5/1 -> Sqrt2/1
  Math Function6/1 -> Add5/2
  Add6/1 -> Math Function6/1
  Product7/1 -> Add6/2
  Trigonometric Function5/1 -> Product7/2
  Add2/1 -> Math Function1/1
  angPos/1 -> Trigonometric Function1/1, Trigonometric Function5/1

== system PTOSim_Lib_UpdatedV3/Motion Conversion/Rotary to Linear Adjustable Rod/Angular to Linear Position/Distance btw flap joint & rod joint along x-axis ==
  Add3 : Sum  Inputs=+-
  Add4 : Sum  Inputs=+-
  Constant4 : Constant  Value=ptosim.rodInit
  Constant5 : Constant  Value=ptosim.crank
  Constant6 : Constant  Value=ptosim.offset
  Math Function2 : Math  Operator=square  SignedPower=on  SaturateOnIntegerOverflow=on
  Math Function3 : Math  Operator=square  SignedPower=on  SaturateOnIntegerOverflow=on
  Sqrt1 : Sqrt  SaturateOnIntegerOverflow=on
  d : Outport
  wires:
  Add3/1 -> Sqrt1/1
  Constant4/1 -> Math Function2/1
  Constant5/1 -> Add4/1
  Constant6/1 -> Add4/2
  Add4/1 -> Math Function3/1
  Math Function3/1 -> Add3/2
  Math Function2/1 -> Add3/1
  Sqrt1/1 -> d/1

== system PTOSim_Lib_UpdatedV3/Motion Conversion/Rotary to Linear Adjustable Rod/Angular to Linear Velocity/Distance btw flap joint & rod joint along x-axis ==
  Add3 : Sum  Inputs=+-
  Add4 : Sum  Inputs=+-
  Constant4 : Constant  Value=ptosim.rodInit
  Constant5 : Constant  Value=ptosim.crank
  Constant6 : Constant  Value=ptosim.offset
  Math Function2 : Math  Operator=square  SignedPower=on  SaturateOnIntegerOverflow=on
  Math Function3 : Math  Operator=square  SignedPower=on  SaturateOnIntegerOverflow=on
  Sqrt1 : Sqrt  SaturateOnIntegerOverflow=on
  d : Outport
  wires:
  Add3/1 -> Sqrt1/1
  Constant4/1 -> Math Function2/1
  Constant5/1 -> Add4/1
  Constant6/1 -> Add4/2
  Add4/1 -> Math Function3/1
  Math Function3/1 -> Add3/2
  Math Function2/1 -> Add3/1
  Sqrt1/1 -> d/1

== system PTOSim_Lib_UpdatedV3/Motion Conversion/Rotary to Linear Adjustable Rod/Angular to Linear Velocity/Subsystem ==
  angPos : Inport
  Add2 : Sum  Inputs=+-
  Add5 : Sum
  Add6 : Sum  Inputs=+-
  Constant2 : Constant  Value=ptosim.crank
  Constant3 : Constant  Value=ptosim.offset
  Constant7 : Constant  Value=ptosim.crank
  Distance btw flap joint & rod joint along x-axis : Subsystem
  Math Function1 : Math  Operator=square  SignedPower=on  SaturateOnIntegerOverflow=on
  Math Function6 : Math  Operator=square  SignedPower=on  SaturateOnIntegerOverflow=on
  Product1 : Product  Inputs=**
  Product7 : Product  Inputs=**
  Sqrt2 : Sqrt  SaturateOnIntegerOverflow=on
  Trigonometric Function1 : Trigonometry  Operator=cos
  Trigonometric Function5 : Trigonometry
  rodLength : Outport
  wires:
  angPos/1 -> Trigonometric Function5/1, Trigonometric Function1/1
  Add2/1 -> Math Function1/1
  Trigonometric Function5/1 -> Product7/2
  Product7/1 -> Add6/2
  Add6/1 -> Math Function6/1
  Math Function6/1 -> Add5/2
  Add5/1 -> Sqrt2/1
  Sqrt2/1 -> rodLength/1
  Constant2/1 -> Product1/1
  Trigonometric Function1/1 -> Product1/2
  Product1/1 -> Add2/1
  Constant3/1 -> Add2/2
  Math Function1/1 -> Add5/1
  Constant7/1 -> Product7/1
  Distance btw flap joint & rod joint along x-axis/1(d) -> Add6/1

== system PTOSim_Lib_UpdatedV3/Motion Conversion/Rotary to Linear Crank/Angular to Linear Position/Initial Distance btw flap joint & crank joint along x-axis ==
  Add3 : Sum  Inputs=+-
  Add4 : Sum  Inputs=+-
  Constant1 : Constant  Value=ptosim.rodLength
  Constant5 : Constant  Value=ptosim.crank
  Constant6 : Constant  Value=ptosim.offset
  Math Function2 : Math  Operator=square  SignedPower=on  SaturateOnIntegerOverflow=on
  Math Function3 : Math  Operator=square  SignedPower=on  SaturateOnIntegerOverflow=on
  Sqrt1 : Sqrt  SaturateOnIntegerOverflow=on
  d : Outport
  wires:
  Add3/1 -> Sqrt1/1
  Constant1/1 -> Math Function2/1
  Constant5/1 -> Add4/1
  Constant6/1 -> Add4/2
  Add4/1 -> Math Function3/1
  Math Function3/1 -> Add3/2
  Math Function2/1 -> Add3/1
  Sqrt1/1 -> d/1

== system PTOSim_Lib_UpdatedV3/Motion Conversion/Rotary to Linear Adjustable Rod/Angle Calculation for PTO/Subsystem1/Distance btw flap joint & rod joint along x-axis ==
  Add3 : Sum  Inputs=+-
  Add4 : Sum  Inputs=+-
  Constant1 : Constant  Value=ptosim.crank
  Constant2 : Constant  Value=ptosim.rodInit
  Constant3 : Constant  Value=ptosim.offset
  Math Function2 : Math  Operator=square  SignedPower=on  SaturateOnIntegerOverflow=on
  Math Function3 : Math  Operator=square  SignedPower=on  SaturateOnIntegerOverflow=on
  Sqrt1 : Sqrt  SaturateOnIntegerOverflow=on
  d : Outport
  wires:
  Sqrt1/1 -> d/1
  Math Function2/1 -> Add3/1
  Math Function3/1 -> Add3/2
  Add4/1 -> Math Function3/1
  Constant3/1 -> Add4/2
  Constant1/1 -> Add4/1
  Constant2/1 -> Math Function2/1
  Add3/1 -> Sqrt1/1

== system PTOSim_Lib_UpdatedV3/Motion Conversion/Rotary to Linear Adjustable Rod/Angle Calculation for PTO/Subsystem2/Distance btw flap joint & rod joint along x-axis ==
  Add3 : Sum  Inputs=+-
  Add4 : Sum  Inputs=+-
  Constant1 : Constant  Value=ptosim.crank
  Constant2 : Constant  Value=ptosim.rodInit
  Constant3 : Constant  Value=ptosim.offset
  Math Function2 : Math  Operator=square  SignedPower=on  SaturateOnIntegerOverflow=on
  Math Function3 : Math  Operator=square  SignedPower=on  SaturateOnIntegerOverflow=on
  Sqrt1 : Sqrt  SaturateOnIntegerOverflow=on
  d : Outport
  wires:
  Sqrt1/1 -> d/1
  Math Function2/1 -> Add3/1
  Math Function3/1 -> Add3/2
  Add4/1 -> Math Function3/1
  Constant3/1 -> Add4/2
  Constant1/1 -> Add4/1
  Constant2/1 -> Math Function2/1
  Add3/1 -> Sqrt1/1
